simulink library "stellaris_lib"  (R2012b)
settings: Solver=ode45  StartTime=0.0  StopTime=10.0  RelTol=1e-3
settings Model: Creator=peselnikmg  LastModifiedBy=peselnikmg

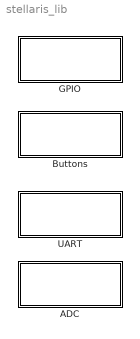
== system stellaris_lib ==
  ADC : Subsystem
  Buttons : Subsystem
  GPIO : Subsystem
  UART : Subsystem

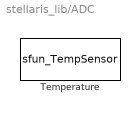
== system stellaris_lib/ADC ==
  Temperature : S-Function  FunctionName=sfun_TempSensor  Parameters=SParameter1  EnableBusSupport=off  mask(Temperature Sensor){SParameter1=Celsius}
      mask prompts: SParameter1 "Units:"
      mask help:
      | This block allows you to read the measurements of internal temperature sensor of TI Stellaris LaunchPad.
      |
      | You should be aware of the following implementation details for this block:
      | 1) Sample sequencer 1 of ADC0 is used (FIFO depth is 4).
      | 2) ADC sample rate is 250 kilo-samples per second.
      | 3) ADC conversion is triggered with software.
      | 4) We wait for ADC conversion to complete in software.
      | 5) We use 64-sample hardware averaging of ADC FIFO.
      settings: AttributesFormatString=%<SParameter1>
      mask TypeOptions SParameter1: Celsius | Fahrenheit
      mask Display: fprintf('Temperature\nSensor');

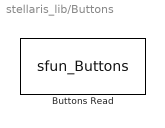
== system stellaris_lib/Buttons ==
  Buttons Read : S-Function  FunctionName=sfun_Buttons  EnableBusSupport=off  mask(Buttons){}
      mask help:
      | This block allows to read values of push buttons SW1 and SW2.
      |
      | The first output is a debounced value (1 sample delay).
      | The second output is a raw value.
      |
      | Both outputs returns bit-packed representation of buttons.
      | Bit 0 corresponds to SW1 and Bit 4 corresponds to SW2.
      | "1" means that the button is pressed,
      | "0" means that the button is not pressed.
      mask Display: fprintf('Buttons')

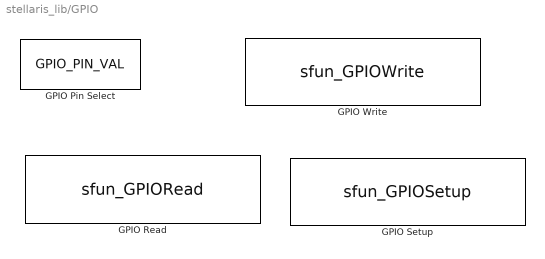
== system stellaris_lib/GPIO ==
  GPIO Pin Select : Constant  Value=GPIO_PIN_VAL  OutDataTypeStr=uint8  LockScale=on  mask(GPIO pin selector){GPIO_PIN_X=GPIO_PIN_0}
      mask prompts: GPIO_PIN_X "Choose GPIO pin:"
      mask help: This block allows to select a specific pin as described in drivers/gpio.h
      mask init:
      | switch GPIO_PIN_X
      |     case 1
      |         GPIO_PIN_VAL = hex2dec('01');
      |     case 2
      |         GPIO_PIN_VAL = hex2dec('02');
      |     case 3
      |         GPIO_PIN_VAL = hex2dec('04');
      |     case 4
      |         GPIO_PIN_VAL = hex2dec('08');
      |     case 5
      |         GPIO_PIN_VAL = hex2dec('10');
      |     case 6
      |         GPIO_PIN_VAL = hex2dec('20');
      |     case 7
      |         GPIO_PIN_VAL = hex2dec('40');
      |     case 8
      |         GPIO_PIN_VAL = hex2dec('80');
      |     otherwise
      |         GPIO_PIN_VAL = hex2dec('01');
      | end
      mask TypeOptions GPIO_PIN_X: GPIO_PIN_0 | GPIO_PIN_1 | GPIO_PIN_2 | GPIO_PIN_3 | GPIO_PIN_4 | GPIO_PIN_5 | GPIO_PIN_6 | GPIO_PIN_7
      mask Display:
      | fprintf('Pin Selector\n\n\n');
      | fprintf('GPIO_PIN_%d',GPIO_PIN_X-1);
  GPIO Read : S-Function  FunctionName=sfun_GPIORead  Parameters=GPIO_PORTVAL_BASE  EnableBusSupport=off  mask(GPIO Read){GPIO_PORTX_BASE=GPIO_PORTF_BASE}
      mask prompts: GPIO_PORTX_BASE "Base Port:"
      mask help:
      | This block allows you to read from GPIO pins.
      | Choose base GPIO port, as defined in inc/hw_memmap.h
      |
      | Input is a bitwise OR of pins you wish to read.
      | Output is a bit-packed value providing the state of specified pins.
      | Any bit that is not specified by input port is returned as a 0. Bits 31:8 should be ignored.
      |
      | You must have GPIO Setup block for the selected port.
      mask init:
      | switch GPIO_PORTX_BASE
      |     case 1 %port A
      |         GPIO_PORTVAL_BASE = hex2dec('40004000');
      |     case 2 %port B
      |         GPIO_PORTVAL_BASE = hex2dec('40005000');
      |     case 3 %port C
      |         GPIO_PORTVAL_BASE = hex2dec('40006000');
      |     case 4 %port D
      |         GPIO_PORTVAL_BASE = hex2dec('40007000');
      |     case 5 %port E
      |         GPIO_PORTVAL_BASE = hex2dec('40024000');
      |     case 6 %port F
      |         GPIO_PORTVAL_BASE = hex2dec('40025000');
      |     otherwise %fallback to port F
      |         GPIO_PORTVAL_BASE = hex2dec('40025000');
      | end
      mask TypeOptions GPIO_PORTX_BASE: GPIO_PORTA_BASE | GPIO_PORTB_BASE | GPIO_PORTC_BASE | GPIO_PORTD_BASE | GPIO_PORTE_BASE | GPIO_PORTF_BASE
      mask Display:
      | fprintf('GPIO Read\n\n\n');
      | fprintf('Base Port: GPIO_PORT%s_BASE',GPIO_PORTX_BASE+64);
  GPIO Setup : S-Function  FunctionName=sfun_GPIOSetup  Parameters=SYSCTL_PERIPH_GPIOVAL,GPIO_PORTVAL_BASE,PinsOutput  EnableBusSupport=off  mask(GPIO Setup){GPIO_PORTX_BASE=GPIO_PORTF_BASE, PinsOutput_0=Input, PinsOutput_1=Output, PinsOutput_2=Output, PinsOutput_3=Output, PinsOutput_4=Input, PinsOutput_5=Input, PinsOutput_6=Input, PinsOutput_7=Input}
      mask prompts: GPIO_PORTX_BASE "Select GPIO Port to configure:"; PinsOutput_0 "Pin 0 is:"; PinsOutput_1 "Pin 1 is:"; PinsOutput_2 "Pin 2 is:"; PinsOutput_3 "Pin 3 is:"; PinsOutput_4 "Pin 4 is:"; PinsOutput_5 "Pin 5 is:"; PinsOutput_6 "Pin 6 is:"; PinsOutput_7 "Pin 7 is:"
      mask help:
      | This block is used to set up (initialize) GPIO port.
      | You need to have as many of these blocks as many ports you wish to initialize.
      |
      | There is no error checking whatsoever. If you add multiple blocks with different parameters for the same port, the behaviour is undefined.
      mask init:
      | switch GPIO_PORTX_BASE
      |     case 1 %port A
      |         GPIO_PORTVAL_BASE = hex2dec('40004000');
      |         SYSCTL_PERIPH_GPIOVAL = hex2dec('20000001');
      |     case 2 %port B
      |         GPIO_PORTVAL_BASE = hex2dec('40005000');
      |         SYSCTL_PERIPH_GPIOVAL = hex2dec('20000002');
      |     case 3 %port C
      |         GPIO_PORTVAL_BASE = hex2dec('40006000');
      |         SYSCTL_PERIPH_GPIOVAL = hex2dec('20000004');
      |     case 4 %port D
      |         GPIO_PORTVAL_BASE = hex2dec('40007000');
      |         SYSCTL_PERIPH_GPIOVAL = hex2dec('20000008');
      |     case 5 %port E
      |         GPIO_PORTVAL_BASE = hex2dec('40024000');
      |         SYSCTL_PERIPH_GPIOVAL = hex2dec('20000010');
      |     case 6 %port F
      |         GPIO_PORTVAL_BASE = hex2dec('40025000');
      |         SYSCTL_PERIPH_GPIOVAL = hex2dec('20000020');
      |     otherwise %fallback to port F
      |         GPIO_PORTVAL_BASE = hex2dec('40025000');
      |         SYSCTL_PERIPH_GPIOVAL = hex2dec('20000020');
      | end
      | 
      | PinsOutput = 0;
      | for i = 1:8
      |     if eval(['PinsOutput_',num2str(i-1)]) == 2
      |         PinsOutput = bitset(PinsOutput,i);
      |     end
      | end
      mask TypeOptions GPIO_PORTX_BASE: GPIO_PORTA_BASE | GPIO_PORTB_BASE | GPIO_PORTC_BASE | GPIO_PORTD_BASE | GPIO_PORTE_BASE | GPIO_PORTF_BASE
      mask TypeOptions PinsOutput_0: Input | Output
      mask TypeOptions PinsOutput_1: Input | Output
      mask TypeOptions PinsOutput_2: Input | Output
      mask TypeOptions PinsOutput_3: Input | Output
      mask TypeOptions PinsOutput_4: Input | Output
      mask TypeOptions PinsOutput_5: Input | Output
      mask TypeOptions PinsOutput_6: Input | Output
      mask TypeOptions PinsOutput_7: Input | Output
      mask Display:
      | fprintf('GPIO Setup\n\n\n');
      | fprintf('Base Port: GPIO_PORT%s_BASE',GPIO_PORTX_BASE+64);
  GPIO Write : S-Function  FunctionName=sfun_GPIOWrite  Parameters=GPIO_PORTVAL_BASE  EnableBusSupport=off  mask(GPIO Write){GPIO_PORTX_BASE=GPIO_PORTF_BASE}
      mask prompts: GPIO_PORTX_BASE "Base Port:"
      mask help:
      | This block allows you to write to GPIO pins.
      | Choose base GPIO port, as defined in inc/hw_memmap.h
      |
      | First input is a bitwise OR of pins you wish to write.
      | Second input is the bit-packed value you wish to write to these pins.
      |
      | You must have GPIO Setup block for the selected port.
      mask init: same as stellaris_lib/GPIO/GPIO Read
      mask TypeOptions GPIO_PORTX_BASE: GPIO_PORTA_BASE | GPIO_PORTB_BASE | GPIO_PORTC_BASE | GPIO_PORTD_BASE | GPIO_PORTE_BASE | GPIO_PORTF_BASE
      mask Display:
      | fprintf('GPIO Write\n\n\n');
      | fprintf('Base Port: GPIO_PORT%s_BASE',GPIO_PORTX_BASE+64);

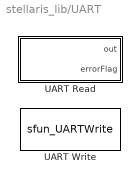
== system stellaris_lib/UART ==
  UART Read : Subsystem  mask(UART Read){nbFlag=on}
      mask prompts: nbFlag "Enable non-blocking mode"
      mask help:
      | This block allows you to data read from UART.
      |
      | First output is data read, cast to int32.
      | Second output is error flag, if non-blocking mode is enabled.
      |
      | In non-blocking mode, if the read buffer is empty, the block outputs the previous value (first output port) and error flag is active (second output port).
      |
      | The baud rate is fixed at 115200.
      | COM port number is defined during installation and can be found using
      | getpref('stellaris','COMPort').
      mask init:
      | if nbFlag
      |     % Terminator -> Outport
      |     if isempty(find_system(gcb,'FollowLinks','on','LookUnderMasks','on','BlockType','Outport','Name','errorFlag'))
      |         % Only replace if there is no Outport block yet
      |         replace_block(gcb,'FollowLinks','on','Name','errorFlag',...
      |         'Outport','noprompt');
      |     end
      | else
      |     % Outport -> Terminator
      |     if isempty(find_system(gcb,'FollowLinks','on','LookUnderMasks','on','BlockType','Terminator'))
      |         % Only replace if there is no Terminator block yet
      |         replace_block(gcb,'FollowLinks','on','Name','errorFlag',...
      |         'Terminator','noprompt');
      |     end
      | end
      mask Display: fprintf('UART Read');
  UART Write : S-Function  FunctionName=sfun_UARTWrite  Parameters=nbFlag  EnableBusSupport=off  mask(UART Write){nbFlag=on}
      mask prompts: nbFlag "Enable non-blocking mode"
      mask help:
      | This block allows you to write data to UART.
      |
      | The baud rate is fixed at 115200.
      | COM port number is defined during installation and can be found using
      | getpref('stellaris','COMPort').
      mask Display: fprintf('UART Write');

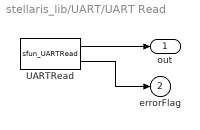
== system stellaris_lib/UART/UART Read ==
  UARTRead : S-Function  FunctionName=sfun_UARTRead  Parameters=nbFlag  EnableBusSupport=off
  out : Outport
  errorFlag : Outport  Port=2
  wires:
  UARTRead/1 -> out/1
  UARTRead/2 -> errorFlag/1
